simulink model "active"  (R2020a)
settings: Solver=ode4  StartTime=0.0  StopTime=40  FixedStep=0.005  RelTol=1e-3
undefined symbols (not defined in the file): A, B, C, D, E, H, K1, K2, params
libraries: simulink x1
settings Model: Creator=aaa  LastModifiedBy=lwb
settings DebuggingCC: UnconnectedInputMsg=none  UnconnectedOutputMsg=none  UnconnectedLineMsg=none
settings ModelReferenceCC: EnableRefExpFcnMdlSchedulingChecks=off
settings RTWCC: Description=Generic Real-Time Target

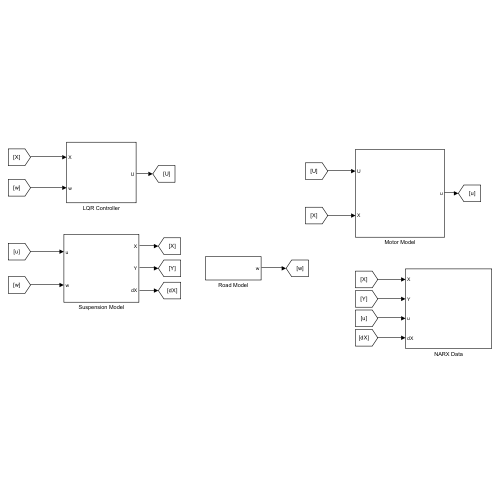
[thumbnail: Simulink's stored preview of the top-level diagram]
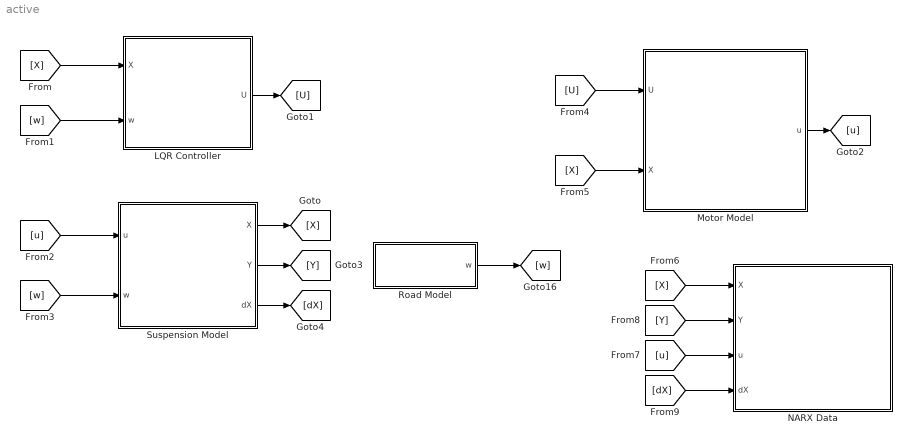
== system active ==
  LQR Controller : Subsystem
  Motor Model : Subsystem
  NARX Data : Subsystem
  Road Model : Subsystem
  Suspension Model : Subsystem
  wires:
  [w] -> Suspension Model/2(w)
  LQR Controller/1(U) -> [U]
  [u] -> Suspension Model/1(u)
  Suspension Model/1(X) -> [X]
  Road Model/1(w) -> [w]
  [w] -> LQR Controller/2(w)
  [X] -> LQR Controller/1(X)
  [U] -> Motor Model/1(U)
  [X] -> Motor Model/2(X)
  Motor Model/1(u) -> [u]
  [X] -> NARX Data/1(X)
  [u] -> NARX Data/3(u)
  Suspension Model/2(Y) -> [Y]
  Suspension Model/3(dX) -> [dX]
  [Y] -> NARX Data/2(Y)
  [dX] -> NARX Data/4(dX)

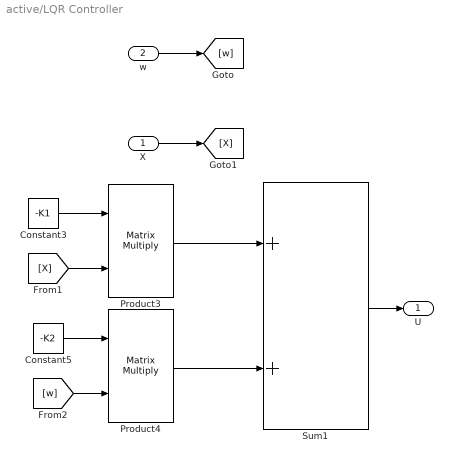
== system active/LQR Controller ==
  X : Inport
  w : Inport  Port=2
  Constant3 : Constant  Value=-K1  VectorParams1D=off
  Constant5 : Constant  Value=-K2  VectorParams1D=off
  Product3 : Product  Multiplication=Matrix(*)
  Product4 : Product  Multiplication=Matrix(*)
  Sum1 : Sum
  U : Outport
  wires:
  [X] -> Product3/2
  Constant5/1 -> Product4/1
  Constant3/1 -> Product3/1
  Sum1/1 -> U/1
  Product3/1 -> Sum1/1
  Product4/1 -> Sum1/2
  [w] -> Product4/2
  w/1 -> [w]
  X/1 -> [X]

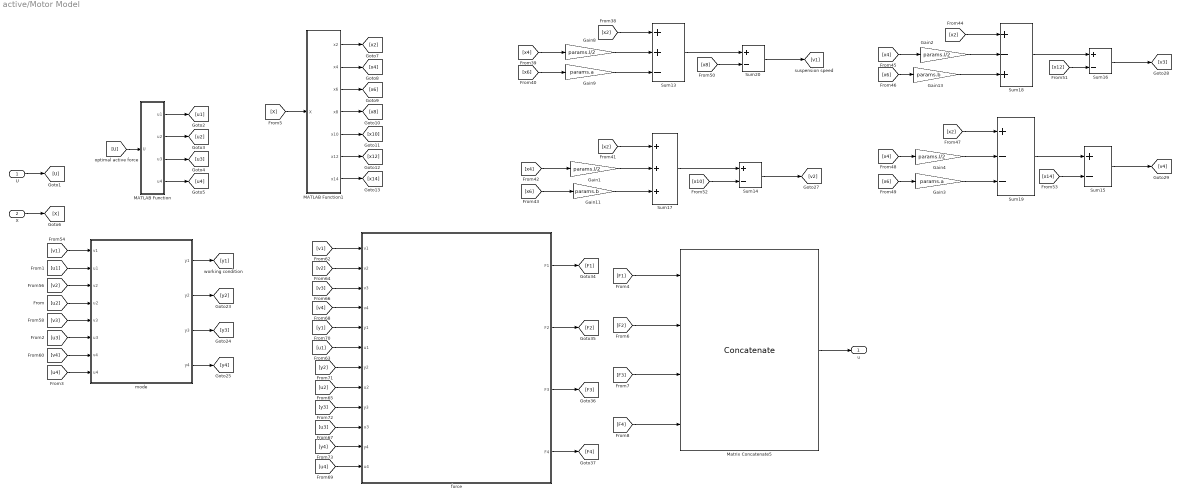
== system active/Motor Model ==
  U : Inport
  X : Inport  Port=2
  Gain{1..2,4,8} (4 alike) : Gain  Gain=params.l/2
  Gain11 : Gain  Gain=params.b
  Gain13 : Gain  Gain=params.b
  Gain3 : Gain  Gain=params.a
  Gain9 : Gain  Gain=params.a
  MATLAB Function : MATLAB Function  TreatAsAtomicUnit=on
  MATLAB Function1 : MATLAB Function  TreatAsAtomicUnit=on
  Matrix Concatenate5 : Concatenate  NumInputs=4  Mode=Multidimensional array
  Sum13 : Sum  Inputs=++-
  Sum{14..16,20} (4 alike) : Sum  Inputs=+-
  Sum17 : Sum  Inputs=+++
  Sum18 : Sum  Inputs=+-+
  Sum19 : Sum  Inputs=+--
  force : Subsystem
  mode : Subsystem
  u : Outport
  wires:
  [y4] -> force/11(y4)
  [u1] -> force/6(u1)
  force/1(F1) -> [F1]
  force/2(F2) -> [F2]
  [v2] -> force/2(v2)
  mode/1(y1) -> [y1]
  [v3] -> force/3(v3)
  [u4] -> mode/8(u4)
  [u3] -> mode/6(u3)
  force/4(F4) -> [F4]
  [v4] -> force/4(v4)
  [y2] -> force/7(y2)
  [v3] -> mode/5(v3)
  mode/2(y2) -> [y2]
  [v4] -> mode/7(v4)
  [u4] -> force/12(u4)
  mode/4(y4) -> [y4]
  [u3] -> force/10(u3)
  mode/3(y3) -> [y3]
  [v2] -> mode/3(v2)
  [u2] -> force/8(u2)
  [v1] -> force/1(v1)
  [v1] -> mode/1(v1)
  [u2] -> mode/4(u2)
  [y3] -> force/9(y3)
  [u1] -> mode/2(u1)
  force/3(F3) -> [F3]
  [y1] -> force/5(y1)
  Sum19/1 -> Sum15/1
  [x14] -> Sum15/2
  Sum16/1 -> [v3]
  [x6] -> Gain13/1
  Gain8/1 -> Sum13/2
  [x2] -> Sum13/1
  Gain1/1 -> Sum17/2
  Sum20/1 -> [v1]
  [x2] -> Sum19/1
  [x4] -> Gain4/1
  [x6] -> Gain9/1
  [x2] -> Sum18/1
  Sum18/1 -> Sum16/1
  Gain9/1 -> Sum13/3
  Sum13/1 -> Sum20/1
  [x12] -> Sum16/2
  Sum15/1 -> [v4]
  Gain3/1 -> Sum19/3
  Gain2/1 -> Sum18/2
  [x4] -> Gain2/1
  [x4] -> Gain1/1
  Gain13/1 -> Sum18/3
  [x6] -> Gain11/1
  Sum17/1 -> Sum14/1
  Gain11/1 -> Sum17/3
  Gain4/1 -> Sum19/2
  [x10] -> Sum14/2
  [x2] -> Sum17/1
  [x4] -> Gain8/1
  Sum14/1 -> [v2]
  [x6] -> Gain3/1
  [x8] -> Sum20/2
  U/1 -> [U]
  [U] -> MATLAB Function/1(U)
  MATLAB Function/2(u2) -> [u2]
  MATLAB Function/3(u3) -> [u3]
  MATLAB Function/4(u4) -> [u4]
  MATLAB Function/1(u1) -> [u1]
  X/1 -> [X]
  [X] -> MATLAB Function1/1(X)
  MATLAB Function1/1(x2) -> [x2]
  MATLAB Function1/2(x4) -> [x4]
  MATLAB Function1/3(x6) -> [x6]
  MATLAB Function1/4(x8) -> [x8]
  MATLAB Function1/5(x10) -> [x10]
  MATLAB Function1/6(x12) -> [x12]
  MATLAB Function1/7(x14) -> [x14]
  [F1] -> Matrix Concatenate5/1
  [F3] -> Matrix Concatenate5/3
  [F4] -> Matrix Concatenate5/4
  [F2] -> Matrix Concatenate5/2
  Matrix Concatenate5/1 -> u/1

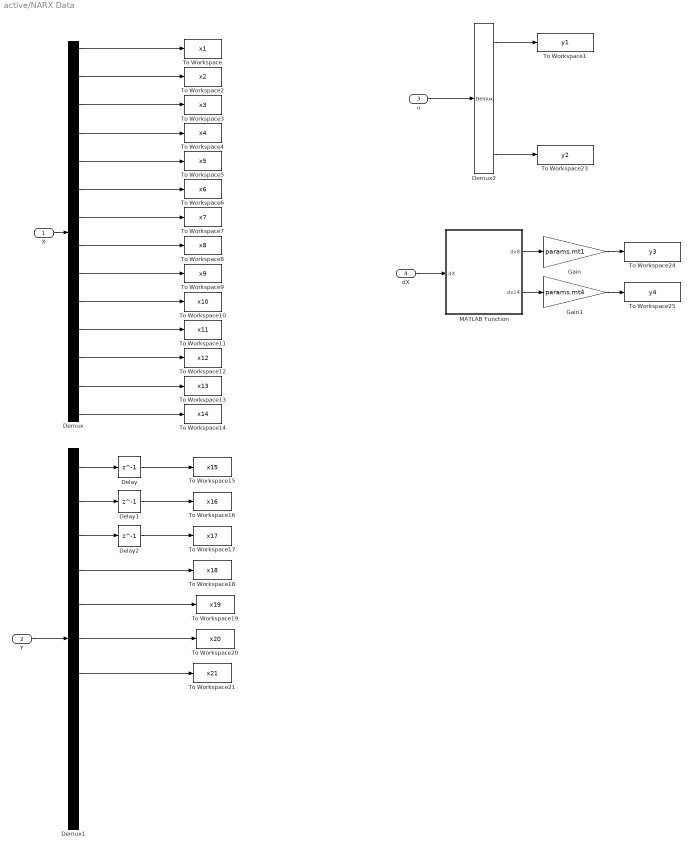
== system active/NARX Data ==
  X : Inport
  Y : Inport  Port=2
  u : Inport  Port=3
  dX : Inport  Port=4
  Delay : Delay  DelayLength=1
  Delay1 : Delay  DelayLength=1
  Delay2 : Delay  DelayLength=1
  Demux : Demux  Outputs=14
  Demux1 : Demux  Outputs=11
  Demux2 : Demux
  Gain : Gain  Gain=params.mt1
  Gain1 : Gain  Gain=params.mt4
  MATLAB Function : MATLAB Function  TreatAsAtomicUnit=on
  To Workspace : ToWorkspace  VariableName=x1  SaveFormat=Timeseries  SampleTime=-1
  To Workspace1 : ToWorkspace  VariableName=y1  SaveFormat=Timeseries  SampleTime=-1
  To Workspace10 : ToWorkspace  VariableName=x10  SaveFormat=Timeseries  SampleTime=-1
  To Workspace11 : ToWorkspace  VariableName=x11  SaveFormat=Timeseries  SampleTime=-1
  To Workspace12 : ToWorkspace  VariableName=x12  SaveFormat=Timeseries  SampleTime=-1
  To Workspace13 : ToWorkspace  VariableName=x13  SaveFormat=Timeseries  SampleTime=-1
  To Workspace14 : ToWorkspace  VariableName=x14  SaveFormat=Timeseries  SampleTime=-1
  To Workspace15 : ToWorkspace  VariableName=x15  SaveFormat=Timeseries  SampleTime=-1
  To Workspace16 : ToWorkspace  VariableName=x16  SaveFormat=Timeseries  SampleTime=-1
  To Workspace17 : ToWorkspace  VariableName=x17  SaveFormat=Timeseries  SampleTime=-1
  To Workspace18 : ToWorkspace  VariableName=x18  SaveFormat=Timeseries  SampleTime=-1
  To Workspace19 : ToWorkspace  VariableName=x19  SaveFormat=Timeseries  SampleTime=-1
  To Workspace2 : ToWorkspace  VariableName=x2  SaveFormat=Timeseries  SampleTime=-1
  To Workspace20 : ToWorkspace  VariableName=x20  SaveFormat=Timeseries  SampleTime=-1
  To Workspace21 : ToWorkspace  VariableName=x21  SaveFormat=Timeseries  SampleTime=-1
  To Workspace23 : ToWorkspace  VariableName=y2  SaveFormat=Timeseries  SampleTime=-1
  To Workspace24 : ToWorkspace  VariableName=y3  SaveFormat=Timeseries  SampleTime=-1
  To Workspace25 : ToWorkspace  VariableName=y4  SaveFormat=Timeseries  SampleTime=-1
  To Workspace3 : ToWorkspace  VariableName=x3  SaveFormat=Timeseries  SampleTime=-1
  To Workspace4 : ToWorkspace  VariableName=x4  SaveFormat=Timeseries  SampleTime=-1
  To Workspace5 : ToWorkspace  VariableName=x5  SaveFormat=Timeseries  SampleTime=-1
  To Workspace6 : ToWorkspace  VariableName=x6  SaveFormat=Timeseries  SampleTime=-1
  To Workspace7 : ToWorkspace  VariableName=x7  SaveFormat=Timeseries  SampleTime=-1
  To Workspace8 : ToWorkspace  VariableName=x8  SaveFormat=Timeseries  SampleTime=-1
  To Workspace9 : ToWorkspace  VariableName=x9  SaveFormat=Timeseries  SampleTime=-1
  wires:
  Demux/7 -> To Workspace7/1
  Demux/5 -> To Workspace5/1
  Demux/11 -> To Workspace11/1
  Demux/3 -> To Workspace3/1
  Demux/2 -> To Workspace2/1
  Demux/13 -> To Workspace13/1
  X/1 -> Demux/1
  Demux/6 -> To Workspace6/1
  Demux/12 -> To Workspace12/1
  Demux/4 -> To Workspace4/1
  Demux/1 -> To Workspace/1
  Demux/8 -> To Workspace8/1
  Demux/9 -> To Workspace9/1
  Demux/10 -> To Workspace10/1
  Demux/14 -> To Workspace14/1
  Y/1 -> Demux1/1
  Demux1/1 -> Delay/1
  Demux1/2 -> Delay1/1
  Demux1/3 -> Delay2/1
  Demux1/4 -> To Workspace18/1
  Demux1/5 -> To Workspace19/1
  Demux1/6 -> To Workspace20/1
  Demux1/7 -> To Workspace21/1
  u/1 -> Demux2/1
  Demux2/1 -> To Workspace1/1
  Demux2/4 -> To Workspace23/1
  dX/1 -> MATLAB Function/1(dX)
  MATLAB Function/1(dx8) -> Gain/1
  MATLAB Function/2(dx14) -> Gain1/1
  Gain/1 -> To Workspace24/1
  Gain1/1 -> To Workspace25/1
  Delay/1 -> To Workspace15/1
  Delay1/1 -> To Workspace16/1
  Delay2/1 -> To Workspace17/1

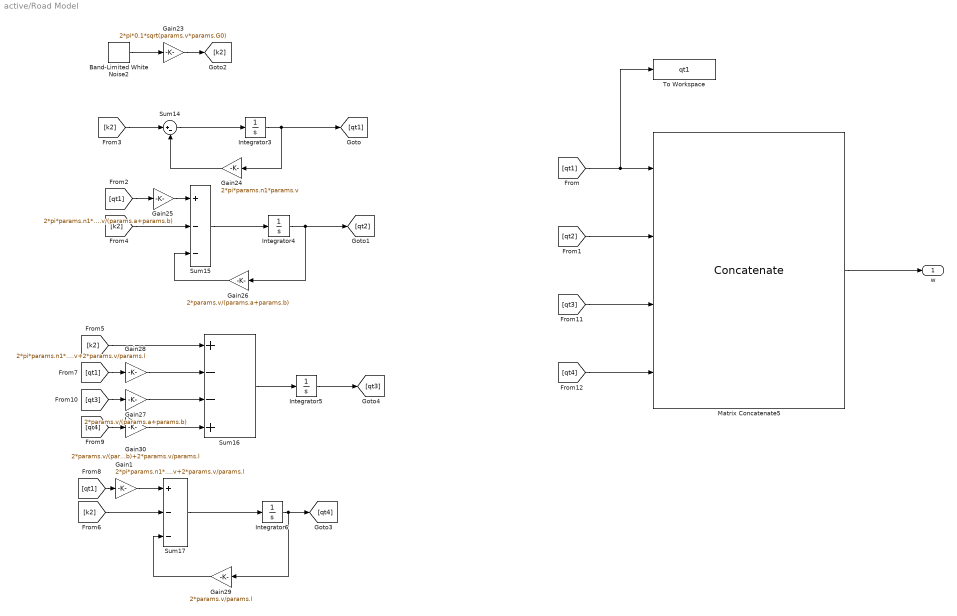
== system active/Road Model ==
  Band-Limited White Noise2 : simulink/Sources/Band-Limited White Noise  Cov=[0.5]  Ts=1/10/params.v  seed=[23341]
  Gain1 : Gain  Gain=2*pi*params.n1*params.v+2*params.v/params.l
  Gain23 : Gain  Gain=2*pi*0.1*sqrt(params.v*params.G0)
  Gain24 : Gain  Gain=2*pi*params.n1*params.v
  Gain25 : Gain  Gain=2*pi*params.n1*params.v+2*params.v/(params.a+params.b)
  Gain26 : Gain  Gain=2*params.v/(params.a+params.b)
  Gain27 : Gain  Gain=2*params.v/(params.a+params.b)
  Gain28 : Gain  Gain=2*pi*params.n1*params.v+2*params.v/params.l
  Gain29 : Gain  Gain=2*params.v/params.l
  Gain30 : Gain  Gain=2*params.v/(params.a+params.b)+2*params.v/params.l
  Integrator{3..6} (4 alike) : Integrator
  Matrix Concatenate5 : Concatenate  NumInputs=4  Mode=Multidimensional array
  Sum14 : Sum  Inputs=|+-
  Sum15 : Sum  Inputs=+--
  Sum16 : Sum  Inputs=+--+
  Sum17 : Sum  Inputs=+--
  To Workspace : ToWorkspace  VariableName=qt1  SaveFormat=Timeseries  SampleTime=-1
  w : Outport
  wires:
  Gain25/1 -> Sum15/1
  Gain27/1 -> Sum16/3
  Gain26/1 -> Sum15/3
  Gain24/1 -> Sum14/2
  Integrator5/1 -> [qt3]
  Integrator3/1 -> Gain24/1, [qt1]
  Matrix Concatenate5/1 -> w/1
  Sum14/1 -> Integrator3/1
  Integrator4/1 -> Gain26/1, [qt2]
  Integrator6/1 -> Gain29/1, [qt4]
  Gain28/1 -> Sum16/2
  Gain29/1 -> Sum17/3
  Sum16/1 -> Integrator5/1
  Sum15/1 -> Integrator4/1
  Gain30/1 -> Sum16/4
  Sum17/1 -> Integrator6/1
  [k2] -> Sum14/1
  Band-Limited White Noise2/1 -> Gain23/1
  Gain23/1 -> [k2]
  [k2] -> Sum15/2
  [k2] -> Sum16/1
  [k2] -> Sum17/2
  [qt1] -> Gain25/1
  [qt1] -> Gain28/1
  [qt1] -> Gain1/1
  Gain1/1 -> Sum17/1
  [qt3] -> Gain27/1
  [qt4] -> Gain30/1
  [qt3] -> Matrix Concatenate5/3
  [qt4] -> Matrix Concatenate5/4
  [qt1] -> To Workspace/1, Matrix Concatenate5/1
  [qt2] -> Matrix Concatenate5/2

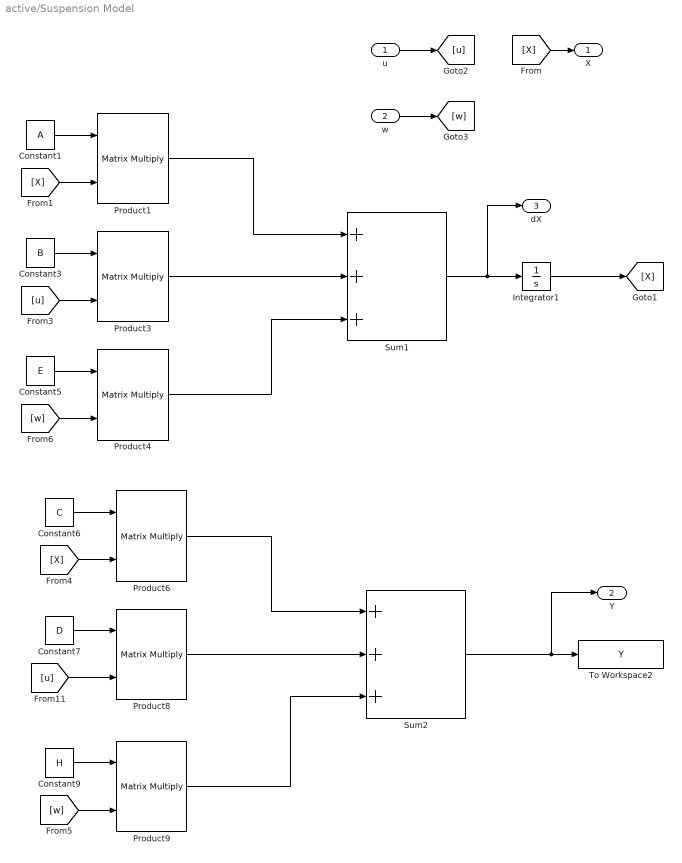
== system active/Suspension Model ==
  u : Inport
  w : Inport  Port=2
  Constant1 : Constant  Value=A  VectorParams1D=off
  Constant3 : Constant  Value=B  VectorParams1D=off
  Constant5 : Constant  Value=E  VectorParams1D=off
  Constant6 : Constant  Value=C  VectorParams1D=off
  Constant7 : Constant  Value=D  VectorParams1D=off
  Constant9 : Constant  Value=H  VectorParams1D=off
  Integrator1 : Integrator
  Product{1,3..4,6,8..9} (6 alike) : Product  Multiplication=Matrix(*)
  Sum1 : Sum  Inputs=+++
  Sum2 : Sum  Inputs=+++
  To Workspace2 : ToWorkspace  VariableName=Y  SaveFormat=Timeseries  SampleTime=-1
  X : Outport
  Y : Outport  Port=2
  dX : Outport  Port=3
  wires:
  Constant3/1 -> Product3/1
  [u] -> Product8/2
  Product4/1 -> Sum1/3
  [u] -> Product3/2
  Product1/1 -> Sum1/1
  Constant1/1 -> Product1/1
  Product6/1 -> Sum2/1
  Sum1/1 -> dX/1, Integrator1/1
  Product9/1 -> Sum2/3
  [X] -> Product1/2
  Product8/1 -> Sum2/2
  Constant7/1 -> Product8/1
  [w] -> Product9/2
  Constant9/1 -> Product9/1
  Constant6/1 -> Product6/1
  Sum2/1 -> Y/1, To Workspace2/1
  Product3/1 -> Sum1/2
  [X] -> Product6/2
  [w] -> Product4/2
  Constant5/1 -> Product4/1
  u/1 -> [u]
  w/1 -> [w]
  Integrator1/1 -> [X]
  [X] -> X/1

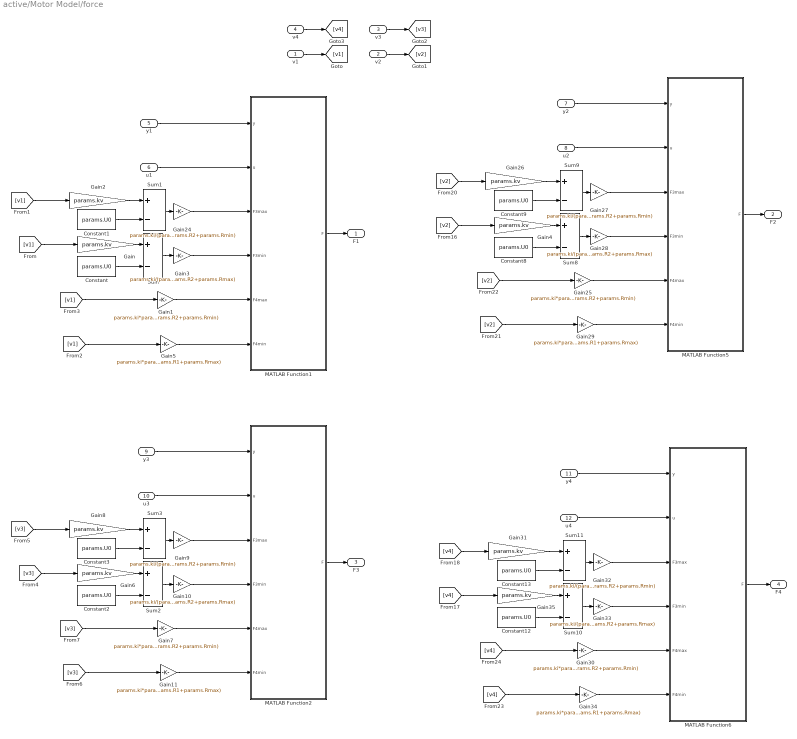
== system active/Motor Model/force ==
  v1 : Inport
  v2 : Inport  Port=2
  v3 : Inport  Port=3
  v4 : Inport  Port=4
  y1 : Inport  Port=5
  u1 : Inport  Port=6
  y2 : Inport  Port=7
  u2 : Inport  Port=8
  y3 : Inport  Port=9
  u3 : Inport  Port=10
  y4 : Inport  Port=11
  u4 : Inport  Port=12
  Constant{,1..3,8..9,12..13} (8 alike) : Constant  Value=params.U0
  Gain{,2,4,6,8,26,31,35} (8 alike) : Gain  Gain=params.kv
  Gain{1,7,25,30} (4 alike) : Gain  Gain=params.ki*params.kv/(params.R2+params.Rmin)
  Gain{3,10,28,33} (4 alike) : Gain  Gain=params.ki/(params.R1+params.R2+params.Rmax)
  Gain{5,11,29,34} (4 alike) : Gain  Gain=params.ki*params.kv/(params.R1+params.Rmax)
  Gain{9,24,27,32} (4 alike) : Gain  Gain=params.ki/(params.R1+params.R2+params.Rmin)
  MATLAB Function1 : MATLAB Function  TreatAsAtomicUnit=on
  MATLAB Function2 : MATLAB Function  TreatAsAtomicUnit=on
  MATLAB Function5 : MATLAB Function  TreatAsAtomicUnit=on
  MATLAB Function6 : MATLAB Function  TreatAsAtomicUnit=on
  Sum{,1..3,8..11} (8 alike) : Sum  Inputs=+-
  F1 : Outport
  F2 : Outport  Port=2
  F3 : Outport  Port=3
  F4 : Outport  Port=4
  wires:
  v4/1 -> [v4]
  Gain3/1 -> MATLAB Function1/4(F3min)
  Gain1/1 -> MATLAB Function1/5(F4max)
  v3/1 -> [v3]
  v2/1 -> [v2]
  [v1] -> Gain1/1
  Gain5/1 -> MATLAB Function1/6(F4min)
  Gain24/1 -> MATLAB Function1/3(F3max)
  [v1] -> Gain/1
  v1/1 -> [v1]
  Constant1/1 -> Sum1/2
  Sum1/1 -> Gain24/1
  Sum/1 -> Gain3/1
  Constant/1 -> Sum/2
  Gain/1 -> Sum/1
  y1/1 -> MATLAB Function1/1(y)
  u1/1 -> MATLAB Function1/2(u)
  [v1] -> Gain2/1
  Gain2/1 -> Sum1/1
  [v1] -> Gain5/1
  MATLAB Function1/1(F) -> F1/1
  MATLAB Function5/1(F) -> F2/1
  [v2] -> Gain29/1
  Gain26/1 -> Sum9/1
  [v2] -> Gain26/1
  u2/1 -> MATLAB Function5/2(u)
  y2/1 -> MATLAB Function5/1(y)
  Gain4/1 -> Sum8/1
  Constant8/1 -> Sum8/2
  Sum8/1 -> Gain28/1
  Sum9/1 -> Gain27/1
  Constant9/1 -> Sum9/2
  [v2] -> Gain4/1
  Gain27/1 -> MATLAB Function5/3(F3max)
  Gain29/1 -> MATLAB Function5/6(F4min)
  [v2] -> Gain25/1
  Gain25/1 -> MATLAB Function5/5(F4max)
  Gain28/1 -> MATLAB Function5/4(F3min)
  MATLAB Function2/1(F) -> F3/1
  [v3] -> Gain11/1
  Gain8/1 -> Sum3/1
  [v3] -> Gain8/1
  u3/1 -> MATLAB Function2/2(u)
  y3/1 -> MATLAB Function2/1(y)
  Gain6/1 -> Sum2/1
  Constant2/1 -> Sum2/2
  Sum2/1 -> Gain10/1
  Sum3/1 -> Gain9/1
  Constant3/1 -> Sum3/2
  [v3] -> Gain6/1
  Gain9/1 -> MATLAB Function2/3(F3max)
  Gain11/1 -> MATLAB Function2/6(F4min)
  [v3] -> Gain7/1
  Gain7/1 -> MATLAB Function2/5(F4max)
  Gain10/1 -> MATLAB Function2/4(F3min)
  Gain33/1 -> MATLAB Function6/4(F3min)
  Gain30/1 -> MATLAB Function6/5(F4max)
  [v4] -> Gain30/1
  Gain34/1 -> MATLAB Function6/6(F4min)
  Gain32/1 -> MATLAB Function6/3(F3max)
  [v4] -> Gain35/1
  Constant13/1 -> Sum11/2
  Sum11/1 -> Gain32/1
  Sum10/1 -> Gain33/1
  Constant12/1 -> Sum10/2
  Gain35/1 -> Sum10/1
  y4/1 -> MATLAB Function6/1(y)
  u4/1 -> MATLAB Function6/2(u)
  [v4] -> Gain31/1
  Gain31/1 -> Sum11/1
  [v4] -> Gain34/1
  MATLAB Function6/1(F) -> F4/1

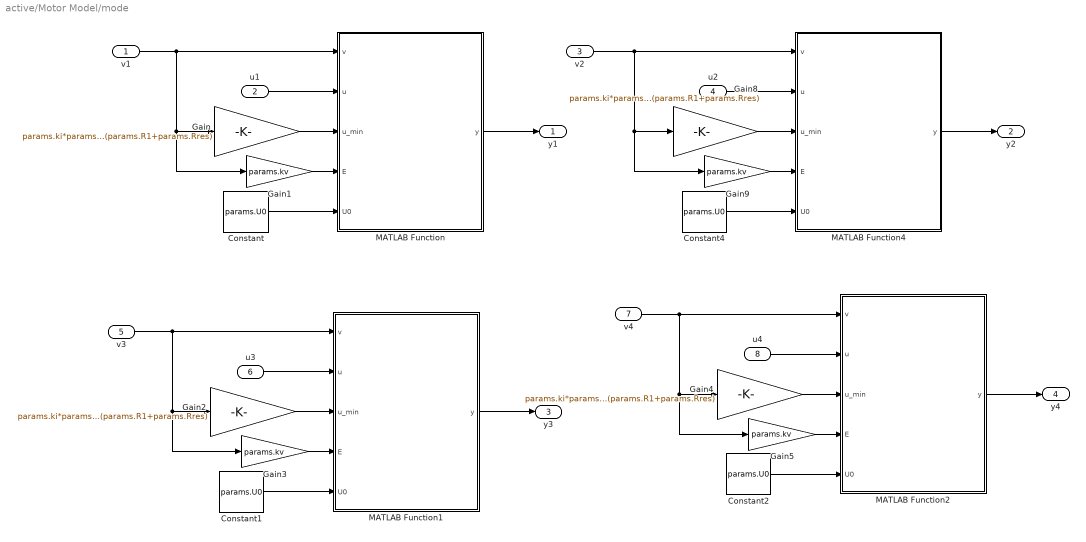
== system active/Motor Model/mode ==
  v1 : Inport
  u1 : Inport  Port=2
  v2 : Inport  Port=3
  u2 : Inport  Port=4
  v3 : Inport  Port=5
  u3 : Inport  Port=6
  v4 : Inport  Port=7
  u4 : Inport  Port=8
  Constant{,1..2,4} (4 alike) : Constant  Value=params.U0
  Gain{,2,4,8} (4 alike) : Gain  Gain=params.ki*params.kv/(params.R1+params.Rres)
  Gain{1,3,5,9} (4 alike) : Gain  Gain=params.kv
  MATLAB Function : MATLAB Function  TreatAsAtomicUnit=on
  MATLAB Function1 : MATLAB Function  TreatAsAtomicUnit=on
  MATLAB Function2 : MATLAB Function  TreatAsAtomicUnit=on
  MATLAB Function4 : MATLAB Function  TreatAsAtomicUnit=on
  y1 : Outport
  y2 : Outport  Port=2
  y3 : Outport  Port=3
  y4 : Outport  Port=4
  wires:
  v1/1 -> MATLAB Function/1(v), Gain1/1, Gain/1
  u1/1 -> MATLAB Function/2(u)
  Gain/1 -> MATLAB Function/3(u_min)
  Gain1/1 -> MATLAB Function/4(E)
  Constant/1 -> MATLAB Function/5(U0)
  MATLAB Function/1(y) -> y1/1
  MATLAB Function4/1(y) -> y2/1
  Constant4/1 -> MATLAB Function4/5(U0)
  Gain9/1 -> MATLAB Function4/4(E)
  Gain8/1 -> MATLAB Function4/3(u_min)
  u2/1 -> MATLAB Function4/2(u)
  v2/1 -> Gain8/1, Gain9/1, MATLAB Function4/1(v)
  MATLAB Function1/1(y) -> y3/1
  Constant1/1 -> MATLAB Function1/5(U0)
  Gain3/1 -> MATLAB Function1/4(E)
  Gain2/1 -> MATLAB Function1/3(u_min)
  u3/1 -> MATLAB Function1/2(u)
  v3/1 -> Gain2/1, Gain3/1, MATLAB Function1/1(v)
  v4/1 -> MATLAB Function2/1(v), Gain5/1, Gain4/1
  u4/1 -> MATLAB Function2/2(u)
  Gain4/1 -> MATLAB Function2/3(u_min)
  Gain5/1 -> MATLAB Function2/4(E)
  Constant2/1 -> MATLAB Function2/5(U0)
  MATLAB Function2/1(y) -> y4/1

== matlab function active/Motor Model/force/MATLAB Function2 ==
  data: y input; F output; u input; F3max input; F3min input; F4max input; F4min input
function F = fcn(y, u, F3max, F3min, F4max, F4min)
if y == 1
    F = u;
elseif y == 2
    F = u;
elseif y == 3
    if u > F3max
        F = F3max;
    elseif u < F3min
        F = F3min;
    else
        F = u;
    end
else
    % elseif y==4
    if u > F4max
        F = F4max;
    elseif u < F4min
        F = F4min;
    else
        F = u;
    end
end

== matlab function active/Motor Model/force/MATLAB Function6 ==
  data: y input; F output; u input; F3max input; F3min input; F4max input; F4min input
function F = fcn(y, u, F3max, F3min, F4max, F4min)
if y == 1
    F = u;
elseif y == 2
    F = u;
elseif y == 3
    if u > F3max
        F = F3max;
    elseif u < F3min
        F = F3min;
    else
        F = u;
    end
else
    % elseif y==4
    if u > F4max
        F = F4max;
    elseif u < F4min
        F = F4min;
    else
        F = u;
    end
end

== matlab function active/NARX Data/MATLAB Function ==
  data: dX input; dx8 output; dx14 output
function [dx8, dx14] = fcn(dX)
dx8 = dX(8);
dx14 = dX(14);

== matlab function active/Motor Model/force/MATLAB Function1 ==
  data: y input; F output; u input; F3max input; F3min input; F4max input; F4min input
function F = fcn(y, u, F3max, F3min, F4max, F4min)
if y == 1
    F = u;
elseif y == 2
    F = u;
elseif y == 3
    if u > F3max
        F = F3max;
    elseif u < F3min
        F = F3min;
    else
        F = u;
    end
else
    % elseif y==4
    if u > F4max
        F = F4max;
    elseif u < F4min
        F = F4min;
    else
        F = u;
    end
end

== matlab function active/Motor Model/MATLAB Function1 ==
  data: X input; x2 output; x4 output; x6 output; x8 output; x10 output; x12 output; x14 output
function [x2, x4, x6, x8, x10, x12, x14] = fcn(X)
x2 = X(2);
x4 = X(4);
x6 = X(6);
x8 = X(8);
x10 = X(10);
x12 = X(12);
x14 = X(14);

== matlab function active/Motor Model/MATLAB Function ==
  data: U input; u1 output; u2 output; u3 output; u4 output
function [u1, u2, u3, u4] = fcn(U)
u1 = U(1);
u2 = U(2);
u3 = U(3);
u4 = U(4);

== matlab function active/Motor Model/mode/MATLAB Function1 ==
  data: v input; u input; y output; u_min input; E input; U0 input
function y = fcn(v, u, u_min, E, U0)
if v * u >= 0
    y = 1;
elseif v * u < 0 && u > u_min
    y = 2;
elseif v * u < 0 && u <= u_min && E > U0
    y = 3;
else
    % elseif v*u<0 && u<=u_min && E<=U0
    y = 4;
end

== matlab function active/Motor Model/mode/MATLAB Function2 ==
  data: v input; u input; y output; u_min input; E input; U0 input
function y = fcn(v, u, u_min, E, U0)
if v * u >= 0
    y = 1;
elseif v * u < 0 && u > u_min
    y = 2;
elseif v * u < 0 && u <= u_min && E > U0
    y = 3;
else
    % elseif v*u<0 && u<=u_min && E<=U0
    y = 4;
end

== matlab function active/Motor Model/force/MATLAB Function5 ==
  data: y input; F output; u input; F3max input; F3min input; F4max input; F4min input
function F = fcn(y, u, F3max, F3min, F4max, F4min)
if y == 1
    F = u;
elseif y == 2
    F = u;
elseif y == 3
    if u > F3max
        F = F3max;
    elseif u < F3min
        F = F3min;
    else
        F = u;
    end
else
    % elseif y==4
    if u > F4max
        F = F4max;
    elseif u < F4min
        F = F4min;
    else
        F = u;
    end
end

== matlab function active/Motor Model/mode/MATLAB Function4 ==
  data: v input; u input; y output; u_min input; E input; U0 input
function y = fcn(v, u, u_min, E, U0)
if v * u >= 0
    y = 1;
elseif v * u < 0 && u > u_min
    y = 2;
elseif v * u < 0 && u <= u_min && E > U0
    y = 3;
else
    % elseif v*u<0 && u<=u_min && E<=U0
    y = 4;
end

== matlab function active/Motor Model/mode/MATLAB Function ==
  data: v input; u input; y output; u_min input; E input; U0 input
function y = fcn(v, u, u_min, E, U0)
if v * u >= 0
    y = 1;
elseif v * u < 0 && u > u_min
    y = 2;
elseif v * u < 0 && u <= u_min && E > U0
    y = 3;
else
    % elseif v*u<0 && u<=u_min && E<=U0
    y = 4;
end
